simulink model "Controltest_gazebo_trajectory_23a"  (R2023a)
settings: Solver=FixedStepAuto  StartTime=0.0  StopTime=15  RelTol=1e-3
StopFcn:
  | figHandles = findobj('Type', 'figure');
  | for i = 1: length(figHandles)
  |     if contains(figHandles(i).Name, 'Sign Following Robot', 'IgnoreCase', true)
  |         close(figHandles(i));
  |     end
  | end
  | 
  | clear figHandles;
model workspace (MAT data in the model file):
  SL_ROS_VariableLengthArrays_MaxSizes.CommonInfo.ArrayTruncateAction = 'EmitWarning'
  SL_ROS_VariableLengthArrays_MaxSizes.MsgTypeMap = containers.Map
  SL_ROS_VariableLengthArrays_MaxSizes.MsgTypeMap.serialization.keys = {'gazebo_msgs/ModelStates', 'sensor_msgs/Image'}
  SL_ROS_VariableLengthArrays_MaxSizes.MsgTypeMap.serialization.values{1}(1).PropertyName = 'Name'
  SL_ROS_VariableLengthArrays_MaxSizes.MsgTypeMap.serialization.values{1}(1).DataType = 'std_msgs/String'
  SL_ROS_VariableLengthArrays_MaxSizes.MsgTypeMap.serialization.values{1}(1).MaxLength = 40
  SL_ROS_VariableLengthArrays_MaxSizes.MsgTypeMap.serialization.values{1}(2).PropertyName = 'Pose'
  SL_ROS_VariableLengthArrays_MaxSizes.MsgTypeMap.serialization.values{1}(2).DataType = 'geometry_msgs/Pose'
  SL_ROS_VariableLengthArrays_MaxSizes.MsgTypeMap.serialization.values{1}(2).MaxLength = 40
  SL_ROS_VariableLengthArrays_MaxSizes.MsgTypeMap.serialization.values{1}(3).PropertyName = 'Twist'
  SL_ROS_VariableLengthArrays_MaxSizes.MsgTypeMap.serialization.values{1}(3).DataType = 'geometry_msgs/Twist'
  SL_ROS_VariableLengthArrays_MaxSizes.MsgTypeMap.serialization.values{1}(3).MaxLength = 40
  SL_ROS_VariableLengthArrays_MaxSizes.MsgTypeMap.serialization.values{2}(1).PropertyName = 'Data'
  SL_ROS_VariableLengthArrays_MaxSizes.MsgTypeMap.serialization.values{2}(1).DataType = 'uint8'
  SL_ROS_VariableLengthArrays_MaxSizes.MsgTypeMap.serialization.values{2}(1).MaxLength = 921600
  SL_ROS_VariableLengthArrays_MaxSizes.MsgTypeMap.serialization.values{2}(2).PropertyName = 'Encoding'
  SL_ROS_VariableLengthArrays_MaxSizes.MsgTypeMap.serialization.values{2}(2).DataType = 'uint8'
  SL_ROS_VariableLengthArrays_MaxSizes.MsgTypeMap.serialization.values{2}(2).MaxLength = 128
  SL_ROS_VariableLengthArrays_MaxSizes.MsgTypeMap.serialization.uniformity = 0
  SL_ROS_VariableLengthArrays_MaxSizes.MsgTypeMap.serialization.keyType = 'char'
  SL_ROS_VariableLengthArrays_MaxSizes.MsgTypeMap.serialization.valueType = 'any'
undefined symbols (not defined in the file or in its folder): Angular, Linear
libraries: robotlib x4, robotgazebolib x1
settings Model: Creator=The MathWorks, Inc.  LastModifiedBy=hugo
settings SolverCC: AlgebraicLoopSolver=TrustRegion
settings OptimizationCC: EnhancedBackFolding=on  PassReuseOutputArgsThreshold=0  MaxStackSize=64  OptimizeBlockOrder=speed  DifferentSizesBufferReuse=on  OptimizationCustomize=off
settings DebuggingCC: ParameterTunabilityLossMsg=error  UnconnectedInputMsg=warning  UnconnectedOutputMsg=warning  UnconnectedLineMsg=warning
settings HardwareCC: ProdBitPerPointer=32  ProdBitPerSizeT=32  ProdBitPerPtrDiffT=32  ProdLargestAtomicFloat=None  ProdIntDivRoundTo=Undefined  ProdEndianess=Unspecified  ProdWordSize=32  ProdHWDeviceType=Generic->Unspecified (assume 32-bit Generic)  UseEmbeddedCoderFeatures=off
settings ModelReferenceCC: EnableRefExpFcnMdlSchedulingChecks=on
settings SFSimCC: MATLABDynamicMemAlloc=off  SimTargetLang=C++
settings RTWCC: Description=Embedded Coder  SystemTargetFile=ert.tlc  HardwareBoard=Robot Operating System (ROS)  TLCOptions="-aInlineSetEventsForThisBaseRateFcn=TLC_FALSE -aSuppressMultiTaskScheduler=TLC_FALSE  -aRateBasedStepFcn=0"  TemplateMakefile=ert_default_tmf  GenerateReport=on  Toolchain=Catkin  LaunchReport=on  TargetLang=C++  DLArmComputeVersion=19.05
settings CodeAppCC: ForceParamTrailComments=on  OperatorAnnotations=on
settings ERTTargetCC: ERTCustomFileBanners=off  SupportContinuousTime=on  SupportNonInlinedSFcns=on  RemoveResetFunc=off  SupportVariableSizeSignals=on  ModelStepFunctionPrototypeControlCompliant=off

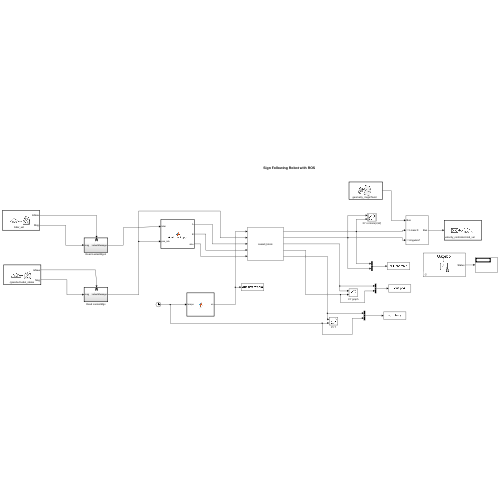
[thumbnail: Simulink's stored preview of the top-level diagram]
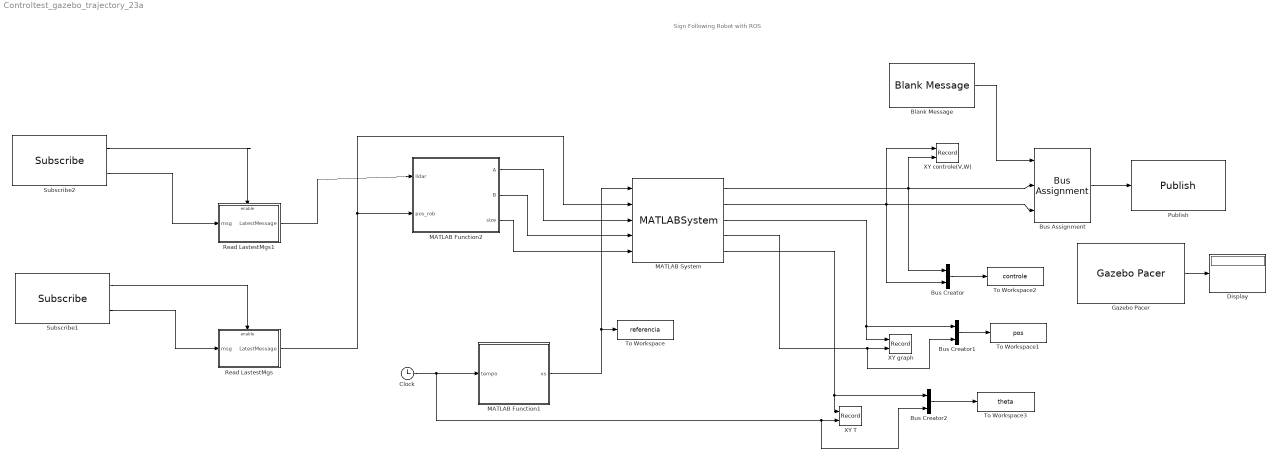
== system Controltest_gazebo_trajectory_23a ==
  note: Sign Following Robot with ROS
  Blank Message : robotlib/Blank Message  messageClass=Message  entityType=geometry_msgs/Twist  messageType=geometry_msgs/Twist  SampleTime=inf  legacyBusStruct=off
  Bus Assignment : BusAssignment  AssignedSignals=Linear.X,Angular.Z
  Bus Creator : BusCreator  Inputs=2
  Bus Creator1 : BusCreator  Inputs=2
  Bus Creator2 : BusCreator  Inputs=2
  Clock : Clock
  Display : Display
  Gazebo Pacer : robotgazebolib/Gazebo Pacer  ResetBehavior=Reset Gazebo simulation time and scene  SampleTime=0.01
  MATLAB Function1 : MATLAB Function  TreatAsAtomicUnit=on
  MATLAB Function2 : MATLAB Function  TreatAsAtomicUnit=on
  MATLAB System : MATLABSystem  System=casadi_block  SimulateUsing=Interpreted execution
      mask Type: casadi_block
      mask Display: disp('casadi_block');
  Publish : robotlib/Publish  topicSource=Select from ROS network  topic=/husky_velocity_controller/cmd_vel  messageType=geometry_msgs/Twist  legacyBusStruct=off  messageQueueLength=1
  Read LastestMgs : Subsystem  TreatAsAtomicUnit=on
  Read LastestMgs1 : Subsystem  TreatAsAtomicUnit=on
  Subscribe1 : robotlib/Subscribe  topicSource=Select from ROS network  topic=/gazebo/model_states  messageType=gazebo_msgs/ModelStates  SampleTime=-1  legacyBusStruct=off  messageQueueLength=1
  Subscribe2 : robotlib/Subscribe  topicSource=Select from ROS network  topic=/lidar_ust  messageType=sensor_msgs/LaserScan  SampleTime=-1  legacyBusStruct=off  messageQueueLength=1
  To Workspace : ToWorkspace  VariableName=referencia  SampleTime=-1
  To Workspace1 : ToWorkspace  VariableName=pos  SaveFormat=Timeseries  SampleTime=-1
  To Workspace2 : ToWorkspace  VariableName=controle  SampleTime=-1
  To Workspace3 : ToWorkspace  VariableName=theta  SaveFormat=Timeseries  SampleTime=-1
  XY T : Record  FileSettingsInternal="{\"entries\":[{\"content\":{\"excelSettings\":{\"content\":{},\"type\":\"Streamout.ExcelSettings\"}},\"type\":\"Streamout.FileSettingStorage\",\"uuid\":\"08c590f7-c346-4c96-8897-3a2789bbd2ac\"}],\"packageUris\":[\"http://schema.mathworks.com/mf0/streamout_blocks/R2020a\"],\"version\":\"1.0\"}"  Layout=[1 1]  SignalsInternal="{\"entries\":[{\"content\":{\"signals\":[{\"content\":{\"blockPath\":[\"Controltest_gazebo_trajectory_23a/XY T\"],\"dimensions\":[1,1],\"domain\":\"Controltest_gazebo_trajectory_23a/XY T\",\"lineColor\":\"#0072bd\",\"plots\":[1],\"port\":1,\"signalID\":50,\"signalName\":\"MATLAB System:5\"},\"type\":\"RecordBlkView.Signal\",\"uuid\":\"0820aadb-c443-4924-9b97-9b3ba3cf0f81\"},{\"content\":{\"blockPath\":[\"Controltest_gazebo_trajectory_23a/XY T\"],\"dimensions\":[1],\"domain\":\"Controltest_gazebo_trajectory_23a/XY T\",\"lineColor\":\"#0072bd\",\"plots\":[1],\"port\":2,\"signalID\":53,\"signalName\":\"Clock\"},\"type\":\"RecordBlkView.Signal\",\"uuid\":\"91aa4ce9-c53a-4398-ac0c-db8bb7633e1d\"}]},\"type\":\"RecordBlkView.InputSignals\",\"uuid\":\"2c9df31d-55b7-4c6f-b319-53ef102db0c6\"}],\"packageUris\":[\"http://schema.mathworks.com/mf0/streamout_blocks/R2020a\"],\"version\":\"1.0\"}"  VisualizationBindings="{\"xyplotplugin\":{\"info\":[{\"series\":[{\"bindingParametersList\":[{\"parameter\":\"X-Axis\",\"signalID\":53,\"signalName\":\"Clock\"},{\"parameter\":\"Y-Axis\",\"signalID\":50,\"signalName\":\"MATLAB System:5\"}],\"seriesID\":10919}],\"subplotID\":1}]}}"  CompatibilityTag=XY
  XY controle(V,W) : Record  FileSettingsInternal="{\"entries\":[{\"content\":{\"excelSettings\":{\"content\":{},\"type\":\"Streamout.ExcelSettings\"}},\"type\":\"Streamout.FileSettingStorage\",\"uuid\":\"66e1edef-69ec-4026-9163-d9525fdf522c\"}],\"packageUris\":[\"http://schema.mathworks.com/mf0/streamout_blocks/R2020a\"],\"version\":\"1.0\"}"  Layout=[1 1]  SignalsInternal="{\"entries\":[{\"content\":{\"signals\":[{\"content\":{\"blockPath\":[\"Controltest_gazebo_trajectory_23a/XY controle(V,W)\"],\"dimensions\":[1,1],\"domain\":\"Controltest_gazebo_trajectory_23a/XY controle(V,W)\",\"lineColor\":\"#fe330a\",\"lineStyle\":\"DASH_DOT\",\"plots\":[1],\"port\":1,\"signalID\":42,\"signalName\":\"MATLAB System:1\"},\"type\":\"RecordBlkView.Signal\",\"uuid\":\"6c214df6-307e-459d-9201-38e894a84124\"},{\"content\":{\"blockPath\":[\"Controltest_gazebo_trajectory_23a/XY controle(V,W)\"],\"dimensions\":[1,1],\"domain\":\"Controltest_gazebo_trajectory_23a/XY controle(V,W)\",\"lineColor\":\"#64d413\",\"lineStyle\":\"DASHED\",\"port\":2,\"signalID\":45,\"signalName\":\"MATLAB System:2\"},\"type\":\"RecordBlkView.Signal\",\"uuid\":\"e2f4b012-a7e5-43c2-8758-91a388ea5904\"}]},\"type\":\"RecordBlkView.InputSignals\",\"uuid\":\"75e9a52c-2012-4acc-9cfa-b96e6e879e38\"}],\"packageUris\":[\"http://schema.mathworks.com/mf0/streamout_blocks/R2020a\"],\"version\":\"1.0\"}"  VisualizationBindings="{\"xyplotplugin\":{\"info\":[{\"series\":[{\"bindingParametersList\":[{\"parameter\":\"X-Axis\",\"signalID\":42,\"signalName\":\"MATLAB System:1\"},{\"parameter\":\"Y-Axis\",\"signalID\":42,\"signalName\":\"MATLAB System:1\"}],\"seriesID\":46825}],\"subplotID\":1}]}}"  CompatibilityTag=XY
  XY graph : Record  FileSettingsInternal="{\"entries\":[{\"content\":{\"excelSettings\":{\"content\":{},\"type\":\"Streamout.ExcelSettings\"}},\"type\":\"Streamout.FileSettingStorage\",\"uuid\":\"42474f06-c070-4592-bb02-3f07125fc3a0\"}],\"packageUris\":[\"http://schema.mathworks.com/mf0/streamout_blocks/R2020a\"],\"version\":\"1.0\"}"  Layout=[1 1]  SignalsInternal="{\"entries\":[{\"content\":{\"signals\":[{\"content\":{\"blockPath\":[\"Controltest_gazebo_trajectory_23a/XY graph\"],\"dimensions\":[1,1],\"domain\":\"Controltest_gazebo_trajectory_23a/XY graph\",\"lineColor\":\"#fe330a\",\"plots\":[1],\"port\":1,\"signalID\":34,\"signalName\":\"MATLAB System:3\"},\"type\":\"RecordBlkView.Signal\",\"uuid\":\"39fa4fd5-e9cf-4131-9dc6-ae51441c72d5\"},{\"content\":{\"blockPath\":[\"Controltest_gazebo_trajectory_23a/XY graph\"],\"dimensions\":[1,1],\"domain\":\"Controltest_gazebo_trajectory_23a/XY graph\",\"lineColor\":\"#64d413\",\"plots\":[1],\"port\":2,\"signalID\":37,\"signalName\":\"MATLAB System:4\"},\"type\":\"RecordBlkView.Signal\",\"uuid\":\"46a36ebc-30c5-452b-a74c-d8875429db3c\"}]},\"type\":\"RecordBlkView.InputSignals\",\"uuid\":\"17f06fc6-7c65-4827-ac91-e8b5d191e4bd\"}],\"packageUris\":[\"http://schema.mathworks.com/mf0/streamout_blocks/R2020a\"],\"version\":\"1.0\"}"  VisualizationBindings="{\"xyplotplugin\":{\"info\":[{\"series\":[{\"bindingParametersList\":[{\"parameter\":\"X-Axis\",\"signalID\":34,\"signalName\":\"MATLAB System:3\"},{\"parameter\":\"Y-Axis\",\"signalID\":37,\"signalName\":\"MATLAB System:4\"}],\"seriesID\":21982}],\"subplotID\":1}]}}"  CompatibilityTag=XY
  wires:
  Bus Assignment/1 -> Publish/1
  Blank Message/1 -> Bus Assignment/1
  Gazebo Pacer/1 -> Display/1
  Clock/1 -> Bus Creator2/2, XY T/2, MATLAB Function1/1(tempo)
  MATLAB Function1/1(xs) -> To Workspace/1, MATLAB System/1
  MATLAB System/1 -> XY controle(V,W)/2, Bus Assignment/2, Bus Creator/1
  MATLAB System/2 -> Bus Creator/2, Bus Assignment/3, XY controle(V,W)/1
  Subscribe1/2 -> Read LastestMgs/1(msg)
  Subscribe1/1 -> Read LastestMgs/Enable
  Read LastestMgs/1(LatestMessage) -> MATLAB Function2/2(pos_rob), MATLAB System/2
  Bus Creator/1 -> To Workspace2/1
  MATLAB System/4 -> Bus Creator1/2, XY graph/2
  MATLAB System/3 -> Bus Creator1/1, XY graph/1
  MATLAB System/5 -> Bus Creator2/1, XY T/1
  Bus Creator1/1 -> To Workspace1/1
  Bus Creator2/1 -> To Workspace3/1
  Subscribe2/2 -> Read LastestMgs1/1(msg)
  Subscribe2/1 -> Read LastestMgs1/Enable
  Read LastestMgs1/1(LatestMessage) -> MATLAB Function2/1(lidar)
  MATLAB Function2/1(A) -> MATLAB System/3
  MATLAB Function2/2(B) -> MATLAB System/4
  MATLAB Function2/3(size) -> MATLAB System/5

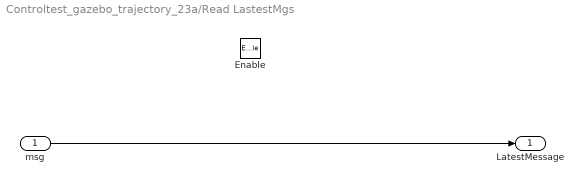
== system Controltest_gazebo_trajectory_23a/Read LastestMgs ==
  msg : Inport
  Enable : EnablePort
  LatestMessage : Outport
  wires:
  msg/1 -> LatestMessage/1

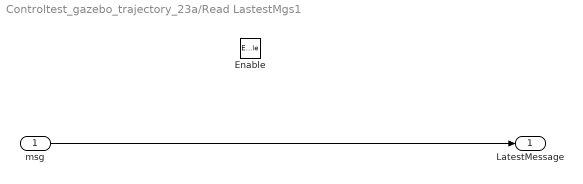
== system Controltest_gazebo_trajectory_23a/Read LastestMgs1 ==
  msg : Inport
  Enable : EnablePort
  LatestMessage : Outport
  wires:
  msg/1 -> LatestMessage/1

== matlab function Controltest_gazebo_trajectory_23a/MATLAB Function1 ==
  data: tempo input; xs output
function xs = fcn(tempo)


% Rastreio de tranjetória em linha reta xd=v*t;yd=1;

xs=[5 5 0]';

== matlab function Controltest_gazebo_trajectory_23a/MATLAB Function2 ==
  data: lidar input; A output; B output; pos_rob input; size output
function [A,B,size] = Matriz_Politopos(lidar,pos_rob)
%#codegen

%% Variaveis globais
epsilon = 0.67;
min_pts = 3;
A_final = [];
b_final = [];
size_matrix = [];

% Receive the data
lidar_msg = receive(lidar);
rob_msg = receive(pos_rob);

%Extract the data from the lidar
ranges = lidar_msg.Ranges; % Extract range data
angles = linspace(lidar_msg.AngleMin, lidar_msg.AngleMax, length(ranges))'; % Calculate angles

% Define the robot's position (x, y) and orientation
robotPos = rob_msg.Pose(37,1).Position; % Example position in 2D
posx = robotPos.X;
posy = robotPos.Y;

%Orientation of the robot
orientation = rob_msg.Pose(37,1).Orientation;
q = [orientation.W, orientation.X, orientation.Y, orientation.Z];
yaw = quat2eul(q);  % Convert quaternion to Euler angles and extract yaw
R_polytope = [cos(yaw(3)) -sin(yaw(3));...
             sin(yaw(3)) cos(yaw(3))];

% Convert ranges to Cartesian coordinates
x = ranges .* cos(angles + yaw(1)) + posx;
y = ranges .* sin(angles + yaw(1)) + posy;

x(isinf(x)) = [];
y(isinf(y)) = [];
%Pontos = double(validPoints);

%%
Pxy = [x,y];
idx = dbscan(Pxy,epsilon,min_pts);

% Unique cluster labels
uniqueLabels = unique(idx); %creates a unique label for each cluster


%% Generate the convex hull for each cluster
for i = 1:length(uniqueLabels)
    clusterLabel = uniqueLabels(i);
    if clusterLabel == -1
        % Skip noise points
        continue;
    end
    % Extract points belonging to the current cluster
    clusterPoints = double(Pxy(idx == clusterLabel, :));

    % Compute the convex hull
    K = convhull(clusterPoints(:,1), clusterPoints(:,2));

    %Get the hull points to generate the matrixes
    hull_points = clusterPoints(K,:);

    % Calculate the half-space representation
    % Each edge of the convex hull defines a half-space
    num_edges = length(K) - 1;
    A_matrices = zeros(num_edges, 2);
    b_vectors = zeros(num_edges, 1);


    %% Get the Matrices A and B
    for j = 1:num_edges
        % Get the start and end points of the edge
        p1 = hull_points(j, :);
        p2 = hull_points(mod(j, num_edges) + 1, :);

        % Calculate the line equation coefficients
        a = p2(2) - p1(2); % y2 - y1
        b = p1(1) - p2(1); % x1 - x2
        c = a * p1(1) + b* p1(2); % - (a * x1 + b * y1)

        A_matrices(j, :) = [a, b]; % Store as negative to conform to Ax <= b
        b_vectors(j) = c;           % Store c
    end

    %take the lines with inf or NaN
    A_matrices(any(isinf(A_matrices) | isnan(A_matrices),2), :) = [];
    b_vectors(any(isinf(b_vectors) | isnan(b_vectors),2), :) = [];
    
    A_final = [A_final;A_matrices];
    b_final = [b_final;b_vectors];
    size_matrix = [size_matrix;length(A_matrices)];

end

A = A_matrices;
B = b_vectors;
size = size_matrix;
end
